simulink model "CassieRealTimeSubsystem"  (R2016b)
settings: Solver=FixedStepDiscrete  StartTime=0.0  StopTime=inf  RelTol=1e-3  EnableMultiTasking=on
InitFcn:
  | realTimeInitFcn;
undefined symbols (not defined in the file): CassieParameters, leftLegMedulla, pelvisMedulla, rightLegMedulla
libraries: xpcethercatlib x98, RealTimeLibrary x10, slrtlib x4, simulink x3
(part 2 of 2)

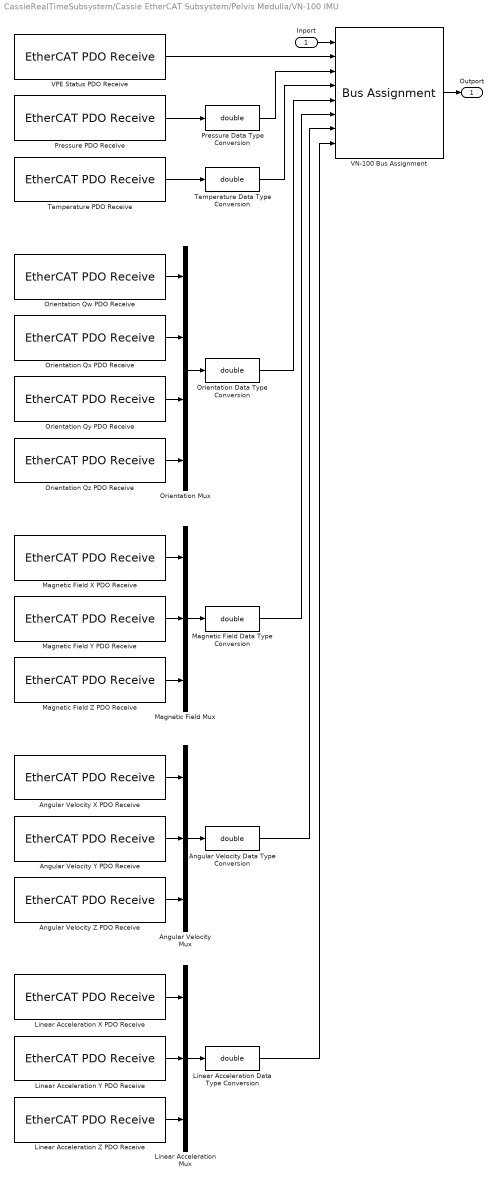
== system CassieRealTimeSubsystem/Cassie EtherCAT Subsystem/Pelvis Medulla/VN-100 IMU ==
  Inport : Inport  LockScale=on
  Angular Velocity Data Type Conversion : DataTypeConversion  OutDataTypeStr=double
  Angular Velocity Mux : Mux  Inputs=3
  Angular Velocity X PDO Receive : xpcethercatlib/EtherCAT PDO Receive  Priority=2  sig_name=Pelvis Medulla.VN Inputs.Angular Velocity X  sig_offset=1168  sig_type=single  type_size=32  sig_dim=1  device_id=0  sample_time=0.000500
  Angular Velocity Y PDO Receive : xpcethercatlib/EtherCAT PDO Receive  Priority=2  sig_name=Pelvis Medulla.VN Inputs.Angular Velocity Y  sig_offset=1200  sig_type=single  type_size=32  sig_dim=1  device_id=0  sample_time=0.000500
  Angular Velocity Z PDO Receive : xpcethercatlib/EtherCAT PDO Receive  Priority=2  sig_name=Pelvis Medulla.VN Inputs.Angular Velocity Z  sig_offset=1232  sig_type=single  type_size=32  sig_dim=1  device_id=0  sample_time=0.000500
  Linear Acceleration Data Type Conversion : DataTypeConversion  OutDataTypeStr=double
  Linear Acceleration Mux : Mux  Inputs=3
  Linear Acceleration X PDO Receive : xpcethercatlib/EtherCAT PDO Receive  Priority=2  sig_name=Pelvis Medulla.VN Inputs.Linear Acceleration X  sig_offset=1264  sig_type=single  type_size=32  sig_dim=1  device_id=0  sample_time=0.000500
  Linear Acceleration Y PDO Receive : xpcethercatlib/EtherCAT PDO Receive  Priority=2  sig_name=Pelvis Medulla.VN Inputs.Linear Acceleration Y  sig_offset=1296  sig_type=single  type_size=32  sig_dim=1  device_id=0  sample_time=0.000500
  Linear Acceleration Z PDO Receive : xpcethercatlib/EtherCAT PDO Receive  Priority=2  sig_name=Pelvis Medulla.VN Inputs.Linear Acceleration Z  sig_offset=1328  sig_type=single  type_size=32  sig_dim=1  device_id=0  sample_time=0.000500
  Magnetic Field Data Type Conversion : DataTypeConversion  OutDataTypeStr=double
  Magnetic Field Mux : Mux  Inputs=3
  Magnetic Field X PDO Receive : xpcethercatlib/EtherCAT PDO Receive  Priority=2  sig_name=Pelvis Medulla.VN Inputs.Magnetic Field X  sig_offset=1360  sig_type=single  type_size=32  sig_dim=1  device_id=0  sample_time=0.000500
  Magnetic Field Y PDO Receive : xpcethercatlib/EtherCAT PDO Receive  Priority=2  sig_name=Pelvis Medulla.VN Inputs.Magnetic Field Y  sig_offset=1392  sig_type=single  type_size=32  sig_dim=1  device_id=0  sample_time=0.000500
  Magnetic Field Z PDO Receive : xpcethercatlib/EtherCAT PDO Receive  Priority=2  sig_name=Pelvis Medulla.VN Inputs.Magnetic Field Z  sig_offset=1424  sig_type=single  type_size=32  sig_dim=1  device_id=0  sample_time=0.000500
  Orientation Data Type Conversion : DataTypeConversion  OutDataTypeStr=double
  Orientation Mux : Mux
  Orientation Qw PDO Receive : xpcethercatlib/EtherCAT PDO Receive  Priority=2  sig_name=Pelvis Medulla.VN Inputs.Orientation Qw  sig_offset=1136  sig_type=single  type_size=32  sig_dim=1  device_id=0  sample_time=0.000500
  Orientation Qx PDO Receive : xpcethercatlib/EtherCAT PDO Receive  Priority=2  sig_name=Pelvis Medulla.VN Inputs.Orientation Qx  sig_offset=1040  sig_type=single  type_size=32  sig_dim=1  device_id=0  sample_time=0.000500
  Orientation Qy PDO Receive : xpcethercatlib/EtherCAT PDO Receive  Priority=2  sig_name=Pelvis Medulla.VN Inputs.Orientation Qy  sig_offset=1072  sig_type=single  type_size=32  sig_dim=1  device_id=0  sample_time=0.000500
  Orientation Qz PDO Receive : xpcethercatlib/EtherCAT PDO Receive  Priority=2  sig_name=Pelvis Medulla.VN Inputs.Orientation Qz  sig_offset=1104  sig_type=single  type_size=32  sig_dim=1  device_id=0  sample_time=0.000500
  Pressure Data Type Conversion : DataTypeConversion  OutDataTypeStr=double
  Pressure PDO Receive : xpcethercatlib/EtherCAT PDO Receive  Priority=2  sig_name=Pelvis Medulla.VN Inputs.Pressure  sig_offset=1488  sig_type=single  type_size=32  sig_dim=1  device_id=0  sample_time=0.000500
  Temperature Data Type Conversion : DataTypeConversion  OutDataTypeStr=double
  Temperature PDO Receive : xpcethercatlib/EtherCAT PDO Receive  Priority=2  sig_name=Pelvis Medulla.VN Inputs.Temperature  sig_offset=1456  sig_type=single  type_size=32  sig_dim=1  device_id=0  sample_time=0.000500
  VN-100 Bus Assignment : BusAssignment  AssignedSignals=pelvisMedulla.vnInputs.vpeStatus,pelvisMedulla.vnInputs.pressure,pelvisMedulla.vnInputs.temperature,pelvisMedulla.vnInputs.orientation,pelvisMedulla.vnInputs.magneticField,pelvisMedulla.vnInputs.angularVelocity,pelvisMedulla.vnInputs.linearAcceleration
  VPE Status PDO Receive : xpcethercatlib/EtherCAT PDO Receive  Priority=2  sig_name=Pelvis Medulla.VN Inputs.VPE Status  sig_offset=1520  sig_type=uint16  type_size=16  sig_dim=1  device_id=0  sample_time=0.000500
  Outport : Outport
  wires:
  VN-100 Bus Assignment/1 -> Outport/1
  Temperature PDO Receive/1 -> Temperature Data Type Conversion/1
  Pressure PDO Receive/1 -> Pressure Data Type Conversion/1
  Inport/1 -> VN-100 Bus Assignment/1
  Linear Acceleration Mux/1 -> Linear Acceleration Data Type Conversion/1
  Angular Velocity Mux/1 -> Angular Velocity Data Type Conversion/1
  Linear Acceleration Y PDO Receive/1 -> Linear Acceleration Mux/2
  Angular Velocity Y PDO Receive/1 -> Angular Velocity Mux/2
  Linear Acceleration X PDO Receive/1 -> Linear Acceleration Mux/1
  Linear Acceleration Z PDO Receive/1 -> Linear Acceleration Mux/3
  Angular Velocity X PDO Receive/1 -> Angular Velocity Mux/1
  Angular Velocity Z PDO Receive/1 -> Angular Velocity Mux/3
  Orientation Mux/1 -> Orientation Data Type Conversion/1
  Orientation Qx PDO Receive/1 -> Orientation Mux/2
  Orientation Qw PDO Receive/1 -> Orientation Mux/1
  Orientation Qy PDO Receive/1 -> Orientation Mux/3
  Orientation Qz PDO Receive/1 -> Orientation Mux/4
  Magnetic Field Mux/1 -> Magnetic Field Data Type Conversion/1
  Magnetic Field Y PDO Receive/1 -> Magnetic Field Mux/2
  Magnetic Field X PDO Receive/1 -> Magnetic Field Mux/1
  Magnetic Field Z PDO Receive/1 -> Magnetic Field Mux/3
  VPE Status PDO Receive/1 -> VN-100 Bus Assignment/2
  Pressure Data Type Conversion/1 -> VN-100 Bus Assignment/3
  Temperature Data Type Conversion/1 -> VN-100 Bus Assignment/4
  Linear Acceleration Data Type Conversion/1 -> VN-100 Bus Assignment/8
  Angular Velocity Data Type Conversion/1 -> VN-100 Bus Assignment/7
  Magnetic Field Data Type Conversion/1 -> VN-100 Bus Assignment/6
  Orientation Data Type Conversion/1 -> VN-100 Bus Assignment/5

== system CassieRealTimeSubsystem/Cassie EtherCAT Subsystem/Right Leg Medulla/Base Medulla ==
  Inport : Inport
  Base Inputs Bus Assignment : BusAssignment  AssignedSignals=rightLegMedulla.baseInputs.cpuLoad,rightLegMedulla.baseInputs.counter
  CPU Load Data Type Conversion : DataTypeConversion  OutDataTypeStr=double
  CPU Load PDO Receive : xpcethercatlib/EtherCAT PDO Receive  Priority=2  sig_name=Right Leg Medulla.Base Inputs.CPU Load  sig_offset=1984  sig_type=uint16  type_size=16  sig_dim=1  device_id=0  sample_time=0.000500
  Counter PDO Receive : xpcethercatlib/EtherCAT PDO Receive  Priority=2  sig_name=Right Leg Medulla.Base Inputs.Counter  sig_offset=1976  sig_type=uint8  type_size=8  sig_dim=1  device_id=0  sample_time=0.000500
  Difference : simulink/Discrete/Difference  ICPrevInput=0.0  OutMin=[]  OutMax=[]  OutDataType=fixdt(1, 16)  OutScaling=2^-10  DoSatur=off
  Outport : Outport
  wires:
  Base Inputs Bus Assignment/1 -> Outport/1
  Counter PDO Receive/1 -> Difference/1
  Difference/1 -> Base Inputs Bus Assignment/3
  Inport/1 -> Base Inputs Bus Assignment/1
  CPU Load PDO Receive/1 -> CPU Load Data Type Conversion/1
  CPU Load Data Type Conversion/1 -> Base Inputs Bus Assignment/2

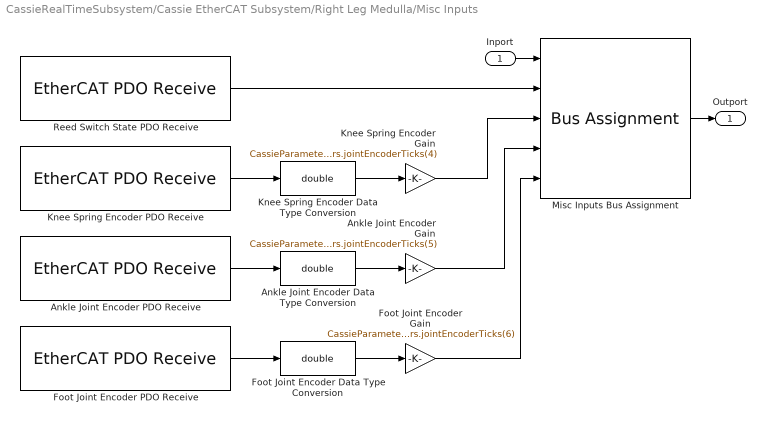
== system CassieRealTimeSubsystem/Cassie EtherCAT Subsystem/Right Leg Medulla/Misc Inputs ==
  Inport : Inport
  Ankle Joint Encoder Data Type Conversion : DataTypeConversion  OutDataTypeStr=double
  Ankle Joint Encoder Gain : Gain  Gain=CassieParameters.jointDirection(5)*2*pi/CassieParameters.jointEncoderTicks(5)
  Ankle Joint Encoder PDO Receive : xpcethercatlib/EtherCAT PDO Receive  Priority=2  sig_name=Right Leg Medulla.Misc Inputs.Ankle Joint Encoder  sig_offset=2032  sig_type=int32  type_size=32  sig_dim=1  device_id=0  sample_time=0.000500
  Foot Joint Encoder Data Type Conversion : DataTypeConversion  OutDataTypeStr=double
  Foot Joint Encoder Gain : Gain  Gain=CassieParameters.jointDirection(6)*2*pi/CassieParameters.jointEncoderTicks(6)
  Foot Joint Encoder PDO Receive : xpcethercatlib/EtherCAT PDO Receive  Priority=2  sig_name=Right Leg Medulla.Misc Inputs.Foot Joint Encoder  sig_offset=2064  sig_type=int32  type_size=32  sig_dim=1  device_id=0  sample_time=0.000500
  Knee Spring Encoder Data Type Conversion : DataTypeConversion  OutDataTypeStr=double
  Knee Spring Encoder Gain : Gain  Gain=CassieParameters.jointDirection(4)*2*pi/CassieParameters.jointEncoderTicks(4)
  Knee Spring Encoder PDO Receive : xpcethercatlib/EtherCAT PDO Receive  Priority=2  sig_name=Right Leg Medulla.Misc Inputs.Knee Spring Encoder  sig_offset=2000  sig_type=int32  type_size=32  sig_dim=1  device_id=0  sample_time=0.000500
  Misc Inputs Bus Assignment : BusAssignment  AssignedSignals=rightLegMedulla.miscInputs.reedSwitchState,rightLegMedulla.miscInputs.kneeSpringEncoder,rightLegMedulla.miscInputs.ankleJointEncoder,rightLegMedulla.miscInputs.footJointEncoder
  Reed Switch State PDO Receive : xpcethercatlib/EtherCAT PDO Receive  Priority=2  sig_name=Right Leg Medulla.Misc Inputs.Reed Switch  sig_offset=2096  sig_type=boolean  type_size=1  sig_dim=1  device_id=0  sample_time=0.000500
  Outport : Outport
  wires:
  Ankle Joint Encoder Data Type Conversion/1 -> Ankle Joint Encoder Gain/1
  Knee Spring Encoder Data Type Conversion/1 -> Knee Spring Encoder Gain/1
  Foot Joint Encoder PDO Receive/1 -> Foot Joint Encoder Data Type Conversion/1
  Foot Joint Encoder Data Type Conversion/1 -> Foot Joint Encoder Gain/1
  Misc Inputs Bus Assignment/1 -> Outport/1
  Knee Spring Encoder PDO Receive/1 -> Knee Spring Encoder Data Type Conversion/1
  Ankle Joint Encoder PDO Receive/1 -> Ankle Joint Encoder Data Type Conversion/1
  Inport/1 -> Misc Inputs Bus Assignment/1
  Reed Switch State PDO Receive/1 -> Misc Inputs Bus Assignment/2
  Knee Spring Encoder Gain/1 -> Misc Inputs Bus Assignment/3
  Ankle Joint Encoder Gain/1 -> Misc Inputs Bus Assignment/4
  Foot Joint Encoder Gain/1 -> Misc Inputs Bus Assignment/5

== matlab function CassieRealTimeSubsystem/Cassie EtherCAT Subsystem/Pelvis Medulla/Battery Management System/ADC to Amperage MATLAB Function ==
  data: adcValue input; A output
function A = adcToAmperage(adcValue) %#codegen
%ADCTOAMPERAGE Convert ADC value to amperage.
%
% Description:
%   The current transducer is connected to the AUXn input channels on the
%   battery monitor chip. In order to get a current reading we have to
%     - Convert the returned ADC value to voltage given the battery
%     monitor specifications
%     - Convert voltage to amperage given the current transducer
%     specifications
%
% Specifications:
%   - Battery Monitor: bq76pl455a-q1
%     - http://www.ti.com/lit/ds/symlink/bq76pl455a-q1.pdf
%     - V_REF = 2.5V
%     - V_AUX = (2*V_REF)/65535*READ_ADC_VALUE
%
%   - Current Transducer: ACS770KCB-150B-PFF-T
%     - sensitivity = 13.3mV/A
%     - sensitivity is negative because current transducer is installed
%     backward on hardware

% Copyright 2017 Mikhail S. Jones

  % Define battery monitor reference voltage for ADC conversion
  V_ref = 2.5;
  
  % Convert battery monitor ADC value to voltage
  V_aux = ((2.*V_ref)./65535).*double(adcValue);
  
  % Define current transducer supply voltage
  if CassieParameters.version == 3
    % Cassie version 3 and 3b
    V_cc = 5.3;
  else
    % Cassie version 1 and 2
    V_cc = 5;
  end % if
  
  % Define current transducer sensitivity with 5V supply voltage
  sensitivity_5V = -13.3/1000;
  
  % Compute adjusted current transducer sensitivity for defined supply
  % voltage
  sensitivity_V_cc = sensitivity_5V*(V_cc/5);
  
  % Convert sensed voltage to corresponding current
  A = (V_aux - V_cc/2)./sensitivity_V_cc;
end % convertToAmperage

== matlab function CassieRealTimeSubsystem/Cassie EtherCAT Subsystem/Pelvis Medulla/Battery Management System/ADC to Celcius MATLAB Function ==
  data: adcValue input; C output
function C = adcToCelcius(adcValue) %#codegen
%ADCTOCELCIUS Convert ADC value to Celcius.
%
% Description:
%   The thermistors are connected to the AUXn input channels on the battery
%   monitor chip. In order to get a temperature reading we have to
%     - Convert the returned ADC value to voltage given the battery
%     monitor specifications
%     - Convert voltage to resistance given the voltage divider circuit
%     on the BMS board
%    - Convert resistance to temperature given the thermistor
%    specifications
%
% Specifications:
%   - Battery Monitor: bq76pl455a-q1
%     - http://www.ti.com/lit/ds/symlink/bq76pl455a-q1.pdf
%     - V_REF = 2.5V
%     - V_AUX = (2*V_REF)/65535*READ_ADC_VALUE
%
%   - Voltage Divider
%     - https://en.wikipedia.org/wiki/Voltage_divider
%     - R_THERM = 10000*(5/V_AUX - 1)
%
%   - Thermistor: BC2647-ND
%     - http://www.vishay.com/docs/29078/ntcle413.pdf
%     - https://en.wikipedia.org/wiki/Thermistor
%     - B = 3435, R0 = 10k, T0 = 298.15 and Rinf = 0.099191
%     - T = B/ln(R/Rinf)

% Copyright 2017 Mikhail S. Jones
  
  V_ref = 2.5;
  V = (2.*V_ref)./65535.*double(adcValue);
  R = 10000.*(5./V - 1);
  K = 3435./log(R./0.099191);
  C = K - 273.15;
end % adcToCelcius

== matlab function CassieRealTimeSubsystem/Cassie EtherCAT Subsystem/Pelvis Medulla/Battery Management System/ADC to Voltage MATLAB Function ==
  data: adcValue input; V output
function V = adcToVoltage(adcValue) %#codegen
%ADCTOVOLTAGE Convert ADC value to voltage.
% 
% Description:
%   The voltage taps are connected to the VSENSE input channels on the
%   battery monitor chip. In order to get a voltage reading we have to
%     - Convert the returned ADC value to voltage given the battery
%     monitor specifications
%
% Specifications:
%   - Battery Monitor: bq76pl455a-q1
%     - http://www.ti.com/lit/ds/symlink/bq76pl455a-q1.pdf
%     - V_REF = 2.5V
%     - V_AUX = (2*V_REF)/65535*READ_ADC_VALUE

% Copyright 2017 Mikhail S. Jones

  V_ref = 2.5;
  V = (2.*V_ref)./65535.*double(adcValue);
end % adcToVoltage

== matlab function CassieRealTimeSubsystem/Cassie EtherCAT Subsystem/Pelvis Medulla/Misc Inputs/ADC to Celcius MATLAB Function ==
  data: adcValue input; C output
function C = adcToCelcius(adcValue)
%ADCTOCELCIUS Convert ADC value to Celcius.
%
% Description:
%   In order to get a temperature reading we have to
%     - Convert the returned ADC value to voltage given the Medulla
%     specifications
%     - Convert voltage to temperature given the Current Multiplier
%     specifications
%
% Specifications:
%   - Medulla: Atmel AT32UC3C
%     - http://www.atmel.com/images/doc32117.pdf
%     - V = 5*READ_ADC_VALUE/4096
%
%   - Power Distribution Board: Vicor VTM48Ex240y012A00
%     - http://cdn.vicorpower.com/documents/datasheets/VTM48EF240T012A00.pdf
%     - C = 20*V

  sensitivity = 20;
  V = 5*(double(adcValue)/4096);
  C = V*sensitivity;
end % adcToCelcius
